simulink library "INT_RailP_VDSync"  (R2016b)
settings: Solver=VariableStepAuto  StartTime=0.0  StopTime=10.0  RelTol=1e-3
settings Model: Creator=zhoutinglin  LastModifiedBy=zhoutinglin

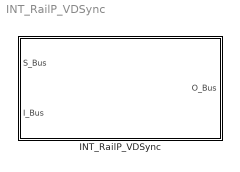
== system INT_RailP_VDSync ==
  INT_RailP_VDSync : Subsystem

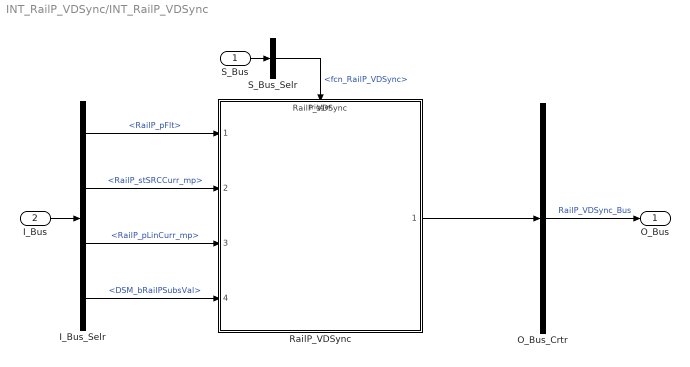
== system INT_RailP_VDSync/INT_RailP_VDSync ==
  S_Bus : Inport
  I_Bus : Inport  Port=2
  I_Bus_Selr : BusSelector  OutputSignals=RailP_pFlt,RailP_stSRCCurr_mp,RailP_pLinCurr_mp,DSM_bRailPSubsVal
  O_Bus_Crtr : BusCreator  Inputs=1
  RailP_VDSync : ModelReference  ModelNameDialog=RailP_VDSync  SimulationMode=Normal  ModelReferenceVersion=1.3  TriggerPortName=function  TriggerPortTriggerType=function-call  TriggerPortStatesWhenEnabling=held
  S_Bus_Selr : BusSelector  OutputSignals=fcn_RailP_VDSync
  O_Bus : Outport
  wires:
  S_Bus_Selr/1 -> RailP_VDSync/Trigger  "<fcn_RailP_VDSync>"
  S_Bus/1 -> S_Bus_Selr/1
  I_Bus/1 -> I_Bus_Selr/1
  I_Bus_Selr/1 -> RailP_VDSync/1  "<RailP_pFlt>"
  I_Bus_Selr/2 -> RailP_VDSync/2  "<RailP_stSRCCurr_mp>"
  I_Bus_Selr/3 -> RailP_VDSync/3  "<RailP_pLinCurr_mp>"
  I_Bus_Selr/4 -> RailP_VDSync/4  "<DSM_bRailPSubsVal>"
  O_Bus_Crtr/1 -> O_Bus/1  "RailP_VDSync_Bus"
  RailP_VDSync/1 -> O_Bus_Crtr/1
